simulink model "spaceShuttleCoCoSim"  (R2017b)
settings: Solver=FixedStepAuto  StartTime=0.0  StopTime=500  FixedStep=0.08  RelTol=1e-3
undefined symbols (not defined in the file or in its folder): sldvsubsys
libraries: MATLAB_Function_lib x2, simulink x2, sldvlib x2
settings Model: Creator=raphael  LastModifiedBy=hbourbou

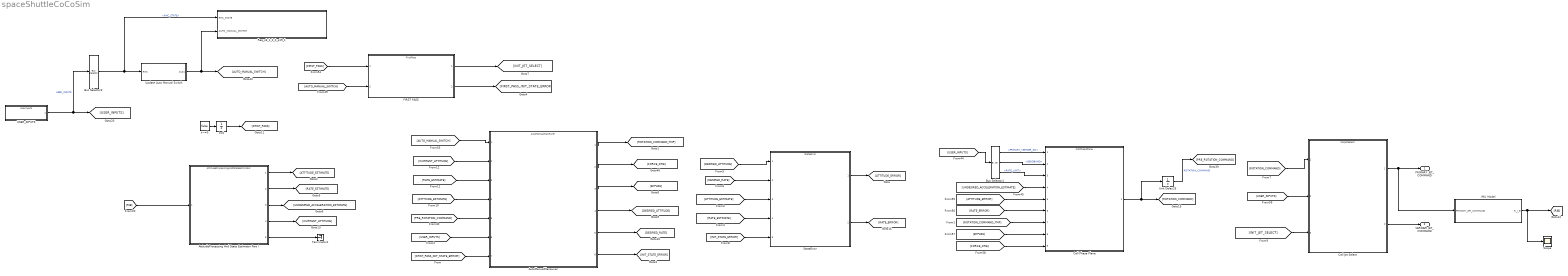
== system spaceShuttleCoCoSim ==
  AttitudeProcessing And State Estimator Part I : ModelReference  ModelNameDialog=AttitudeProcessingANDStateEstimator.slx  SimulationMode=Normal  ModelReferenceVersion=1.45
  AutoManualManeuver : ModelReference  ModelNameDialog=AutoManualManeuver.slx  SimulationMode=Normal  ModelReferenceVersion=1.229
  Bus Selector1 : BusSelector  OutputSignals=PRIMARY_VERNIER_SW,DEADBAND,RATE_LIMIT
  Bus Selector3 : BusSelector  OutputSignals=RHC_STATE
  Call Jet Select : ModelReference  ModelNameDialog=CallJetSelect.slx  SimulationMode=Normal  ModelReferenceVersion=1.34
  Call Phase Plane : ModelReference  ModelNameDialog=CallPhasePlane.slx  SimulationMode=Normal  ModelReferenceVersion=1.10
  FIRST PASS : ModelReference  ModelNameDialog=FirstPass.slx  SimulationMode=Normal  ModelReferenceVersion=1.28
  IMU Model : Subsystem
  Req_s3_1_2_2_p19_1 : Subsystem  Tag=VerificationSubsystem  DisableCoverage=on  LoadFcn=sldvsubsys('check')  TreatAsAtomicUnit=on  SimViewingDevice=on  mask(VerificationSubsystem){}
      mask init:
      | sldvsubsys('maskInit');
      settings: CopyFcn=sldvsubsys('copy');  OpenFcn=open_system(gcb,'force');
      settings: PreSaveFcn=|
      | set_param(gcb,'SimViewingDevice','on');
      | sldvsubsys('check');
      mask Help: helpview(fullfile(docroot,'toolbox','sldv','sldv.map'),'verificationsubsystem')
      mask Display: image(imread('sldvicon_versubsys.png','BackGroundColor',[1 1 1]),'center');
  Scope : Scope
  StateError : ModelReference  ModelNameDialog=StateError.slx  SimulationMode=Normal  ModelReferenceVersion=1.18
  Terminator1 : Terminator
  USER_INPUTS : ModelReference  ModelNameDialog=UserInputs.slx  SimulationMode=Normal  ModelReferenceVersion=1.13
  Unit Delay25 : UnitDelay  InitialCondition=[0;0;0]  SampleTime=-1
  Update Auto Manual Switch : Subsystem
  t=0 : UnitDelay  InitialCondition=true  SampleTime=-1
  t~=0 : Constant  Value=false
  PRIMARY_JET_COMMAND : Outport
  VERNIER_JET_COMMAND : Outport  Port=2
  wires:
  AttitudeProcessing And State Estimator Part I/3 -> [UNDESIRED_ACCELERATION_ESTIMATE]
  IMU Model/1(R_I_B) -> Scope/1, [RIB]
  Call Phase Plane/1 -> [ROTATION_COMMAND], Unit Delay25/1
  Call Jet Select/1 -> IMU Model/1(PRIMARY_JET_COMMAND), PRIMARY_JET_COMMAND/1
  Call Jet Select/2 -> VERNIER_JET_COMMAND/1
  USER_INPUTS/1 -> Bus Selector3/1, [USER_INPUTS]  "USER_INPUTS"
  [USER_INPUTS] -> Bus Selector1/1
  [BYPASS] -> Call Phase Plane/8
  [FORCE_FIRE] -> Call Phase Plane/9
  [RATE_ERROR] -> Call Phase Plane/6
  [ATTITUDE_ERROR] -> Call Phase Plane/5
  [UNDESIRED_ACCELERATION_ESTIMATE] -> Call Phase Plane/4
  Bus Selector1/3 -> Call Phase Plane/3  "<RATE_LIMIT>"
  Bus Selector1/2 -> Call Phase Plane/2  "<DEADBAND>"
  Bus Selector1/1 -> Call Phase Plane/1  "<PRIMARY_VERNIER_SW>"
  Bus Selector3/1 -> Req_s3_1_2_2_p19_1/1(RHC_STATE), Update Auto Manual Switch/1(RHC)  "<RHC_STATE>"
  [ROTATION_COMMAND_TMP] -> Call Phase Plane/7
  AttitudeProcessing And State Estimator Part I/5 -> Terminator1/1
  AutoManualManeuver/1 -> [ROTATION_COMMAND_TMP]
  AutoManualManeuver/2 -> [FORCE_FIRE]
  AutoManualManeuver/3 -> [BYPASS]
  StateError/1 -> [ATTITUDE_ERROR]
  StateError/2 -> [RATE_ERROR]
  AttitudeProcessing And State Estimator Part I/1 -> [ATTITUDE_ESTIMATE]
  AttitudeProcessing And State Estimator Part I/2 -> [RATE_ESTIMATE]
  [AUTO_MANUAL_SWITCH] -> AutoManualManeuver/1
  [PRE_ROTATION_COMMAND] -> AutoManualManeuver/5
  [USER_INPUTS] -> AutoManualManeuver/6
  [ATTITUDE_ESTIMATE] -> StateError/3
  [RATE_ESTIMATE] -> StateError/4
  Unit Delay25/1 -> [PRE_ROTATION_COMMAND]  "ROTATION_COMMAND"
  [USER_INPUTS] -> Call Jet Select/2
  FIRST PASS/2 -> [FIRST_PASS_INIT_STATE_ERROR]
  FIRST PASS/1 -> [INIT_JET_SELECT]
  [FIRST_PASS] -> FIRST PASS/1
  [AUTO_MANUAL_SWITCH] -> FIRST PASS/2
  [FIRST_PASS_INIT_STATE_ERROR] -> AutoManualManeuver/7
  t~=0/1 -> t=0/1
  Update Auto Manual Switch/1(Out1) -> [AUTO_MANUAL_SWITCH], Req_s3_1_2_2_p19_1/2(AUTO_MANUAL_SWITCH)
  t=0/1 -> [FIRST_PASS]
  AutoManualManeuver/4 -> [DESIRED_ATTITUDE]
  [DESIRED_ATTITUDE] -> StateError/1
  AutoManualManeuver/5 -> [DESIRED_RATE]
  [DESIRED_RATE] -> StateError/2
  [ROTATION_COMMAND] -> Call Jet Select/1
  AutoManualManeuver/6 -> [INIT_STATE_ERROR]
  [INIT_STATE_ERROR] -> StateError/5
  [INIT_JET_SELECT] -> Call Jet Select/3
  [ATTITUDE_ESTIMATE] -> AutoManualManeuver/4
  [RATE_ESTIMATE] -> AutoManualManeuver/3
  AttitudeProcessing And State Estimator Part I/4 -> [CURRENT_ATTITUDE]
  [CURRENT_ATTITUDE] -> AutoManualManeuver/2
  [RIB] -> AttitudeProcessing And State Estimator Part I/1

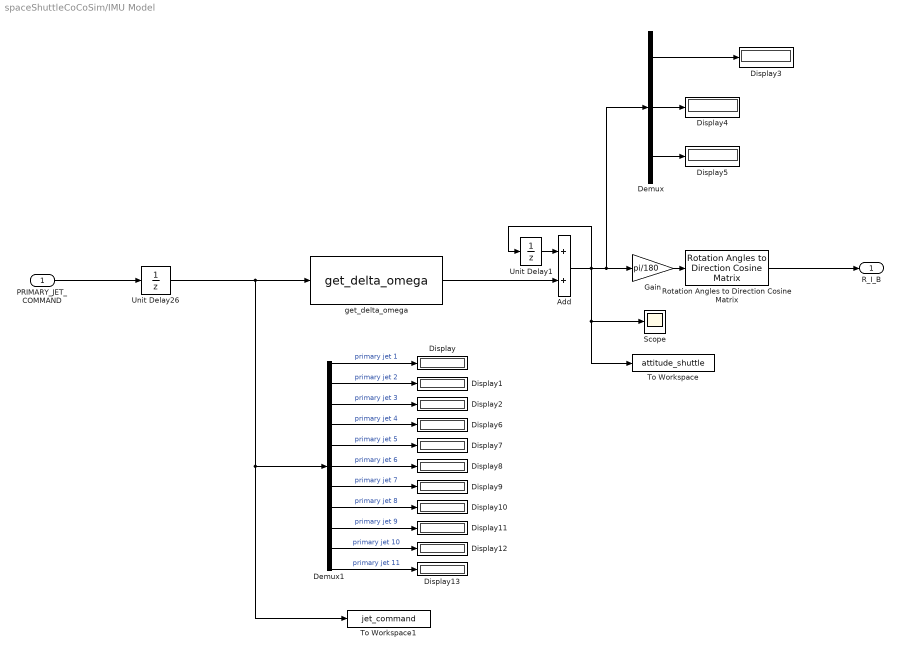
== system spaceShuttleCoCoSim/IMU Model ==
  PRIMARY_JET_COMMAND : Inport
  Add : Sum
  Demux : Demux  Outputs=3
  Demux1 : Demux  Outputs=11
  Display{,1..13} (14 alike) : Display
  Gain : Gain  Gain=pi/180
  Rotation Angles to Direction Cosine Matrix : MATLAB_Function_lib/Rotation Angles to Direction Cosine Matrix
  Scope : Scope
  To Workspace : ToWorkspace  VariableName=attitude_shuttle  SaveFormat=Timeseries  SampleTime=-1
  To Workspace1 : ToWorkspace  VariableName=jet_command  SaveFormat=Timeseries  SampleTime=-1
  Unit Delay1 : UnitDelay  InitialCondition=[50;50;50]  SampleTime=-1
  Unit Delay26 : UnitDelay  InitialCondition=[0;0;0;0;0;0;0;0;0;0;0]  SampleTime=-1
  get_delta_omega : MATLAB_Function_lib/get_delta_omega
  R_I_B : Outport
  wires:
  Gain/1 -> Rotation Angles to Direction Cosine Matrix/1
  Unit Delay1/1 -> Add/1
  Add/1 -> Gain/1, Demux/1, To Workspace/1, Scope/1, Unit Delay1/1
  get_delta_omega/1 -> Add/2
  Demux/3 -> Display5/1
  Demux/2 -> Display4/1
  Demux/1 -> Display3/1
  Demux1/1 -> Display/1  "primary jet 1"
  Demux1/2 -> Display1/1  "primary jet 2"
  Demux1/7 -> Display9/1  "primary jet 7"
  Demux1/6 -> Display8/1  "primary jet 6"
  Demux1/5 -> Display7/1  "primary jet 5"
  Demux1/4 -> Display6/1  "primary jet 4"
  Demux1/3 -> Display2/1  "primary jet 3"
  Demux1/9 -> Display11/1  "primary jet 9"
  Demux1/8 -> Display10/1  "primary jet 8"
  Demux1/10 -> Display12/1  "primary jet 10"
  Demux1/11 -> Display13/1  "primary jet 11"
  Rotation Angles to Direction Cosine Matrix/1 -> R_I_B/1
  PRIMARY_JET_COMMAND/1 -> Unit Delay26/1
  Unit Delay26/1 -> get_delta_omega/1, Demux1/1, To Workspace1/1

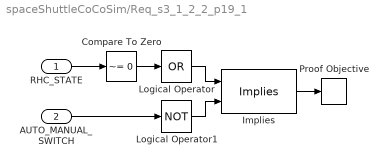
== system spaceShuttleCoCoSim/Req_s3_1_2_2_p19_1 ==
  RHC_STATE : Inport  PortDimensions=3
  AUTO_MANUAL_SWITCH : Inport  Port=2
  Compare To Zero : simulink/Logic and Bit Operations/Compare To Zero  relop=~=  OutDataTypeStr=boolean
  Implies : sldvlib/Verification Utilities/Implies
      settings: SourceProductName=Simulink Design Verifier  SourceProductBaseCode=DV
  Logical Operator : Logic  Operator=OR  Inputs=1  AllPortsSameDT=off  OutDataTypeStr=boolean
  Logical Operator1 : Logic  Operator=NOT  AllPortsSameDT=off  OutDataTypeStr=boolean
  Proof Objective : sldvlib/Objectives and Constraints/Proof Objective  enabled=on  customAVTBlockType=Proof Objective  intervals=true  dispValues=on  outEnabled=off  enableStopSim=off
      settings: AttributesFormatString=%<intervals>  SourceProductName=Simulink Design Verifier  SourceProductBaseCode=DV
  wires:
  RHC_STATE/1 -> Compare To Zero/1
  Compare To Zero/1 -> Logical Operator/1
  Logical Operator/1 -> Implies/1
  AUTO_MANUAL_SWITCH/1 -> Logical Operator1/1
  Implies/1 -> Proof Objective/1
  Logical Operator1/1 -> Implies/2

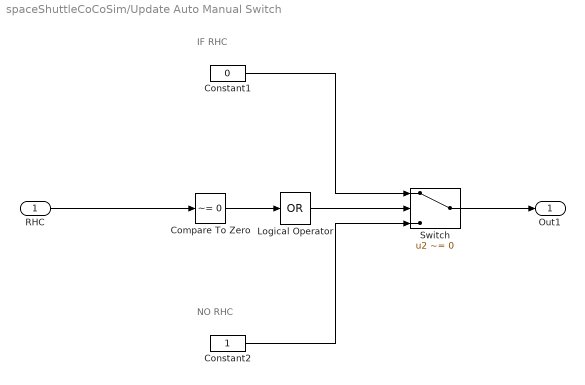
== system spaceShuttleCoCoSim/Update Auto Manual Switch ==
  note: NO RHC
  note: IF RHC
  RHC : Inport
  Compare To Zero : simulink/Logic and Bit Operations/Compare To Zero  relop=~=  OutDataTypeStr=boolean
  Constant1 : Constant  Value=0  OutDataTypeStr=boolean
  Constant2 : Constant  OutDataTypeStr=boolean
  Logical Operator : Logic  Operator=OR  Inputs=1  AllPortsSameDT=off  OutDataTypeStr=boolean
  Switch : Switch  Criteria=u2 ~= 0
  Out1 : Outport
  wires:
  Switch/1 -> Out1/1
  Compare To Zero/1 -> Logical Operator/1
  Logical Operator/1 -> Switch/2
  Constant1/1 -> Switch/1
  RHC/1 -> Compare To Zero/1
  Constant2/1 -> Switch/3
